simulink model "PhysicalEverSimmer"  (R2026a)
settings: Solver=VariableStepAuto  StopTime=14400
undefined symbols (not defined in the file or in its folder): ES_PackRate_bph, ES_PrepRate_bph, ES_QCRate_bph, ES_Resupply_bph, Fault_T_Cell1, Fault_T_Cell2, Fault_T_Cell3, Recipe_Block_s, Recipe_Count, Resupply_Cutoff_T, Transport_Latency_s, Transport_Rate_bph
(part 2 of 2)

== system PhysicalEverSimmer/ProductionCell1/CellCookVat ==
  in_preppedBatch : Inport  PortName=preppedBatch  Element=flow_bps
  in_directive : Inport  Port=2  PortName=directive  Element=setpoint
  En_Gate_Fault_T_Cell1 : Product
  Gate_Fault_T_Cell1 : Step  Time=Fault_T_Cell1  InitialValue=1  FinalValue=0  SampleTime=0
  StateDbl : DataTypeConversion  OutDataTypeStr=double  SaturateOnIntegerOverflow=off  RndMeth=Floor
  ToLitres : Gain  Gain=1800
  Trm37 : Terminator
  Vat : ModelReference  ModelNameDialog=BehCookVat  UsingDefaultArgumentValue=0,0,0,0,0,0,0,0  SimulationMode=Normal  ModelReferenceVersion=1.8
  cookedSoup_c1 : Constant  Value=0
  cookedSoup_c2 : Constant  Value=0
  statusCook_c1 : Constant
  statusCook_c2 : Constant  Value=0
  out_cookedSoup : Outport  PortName=cookedSoup  Element=batchId
  cookedSoup_el2 : Outport  PortName=cookedSoup  Element=volume_L
  cookedSoup_el3 : Outport  PortName=cookedSoup  Element=temp_C
  cookedSoup_el4 : Outport  PortName=cookedSoup  Element=contamination_ppm
  cookedSoup_el5 : Outport  PortName=cookedSoup  Element=flow_bps
  out_statusCook : Outport  Port=2  PortName=statusCook  Element=unitId
  statusCook_el2 : Outport  Port=2  PortName=statusCook  Element=opState
  statusCook_el3 : Outport  Port=2  PortName=statusCook  Element=faultCode
  statusCook_el4 : Outport  Port=2  PortName=statusCook  Element=power_kW
  statusCook_el5 : Outport  Port=2  PortName=statusCook  Element=health
  wires:
  cookedSoup_c2/1 -> cookedSoup_el4/1
  En_Gate_Fault_T_Cell1/1 -> Vat/2
  statusCook_c1/1 -> out_statusCook/1
  in_directive/1 -> En_Gate_Fault_T_Cell1/1
  statusCook_c2/1 -> statusCook_el3/1
  Vat/5 -> Trm37/1
  Gate_Fault_T_Cell1/1 -> En_Gate_Fault_T_Cell1/2, statusCook_el5/1
  cookedSoup_c1/1 -> out_cookedSoup/1
  ToLitres/1 -> cookedSoup_el2/1
  in_preppedBatch/1 -> Vat/1
  Vat/1 -> cookedSoup_el5/1, ToLitres/1
  Vat/2 -> statusCook_el4/1
  Vat/3 -> cookedSoup_el3/1  "vatTemp_Cell1"
  Vat/4 -> StateDbl/1  "vatState_Cell1"
  StateDbl/1 -> statusCook_el2/1

== system PhysicalEverSimmer/ProductionCell1/CellPackager ==
  in_approvedSoup : Inport  PortName=approvedSoup  Element=flow_bps
  in_directive : Inport  Port=2  PortName=directive  Element=setpoint
  En_Gate_Fault_T_Cell1 : Product
  Gate_Fault_T_Cell1 : Step  Time=Fault_T_Cell1  InitialValue=1  FinalValue=0  SampleTime=0
  Pack : ModelReference  ModelNameDialog=BehPackager  UsingDefaultArgumentValue=0,0  SimulationMode=Normal  ModelReferenceVersion=1.4
  PackDraw : Constant  Value=ES_PackRate_bph/3600
  Surge : ModelReference  ModelNameDialog=BehStorage  UsingDefaultArgumentValue=0,0  SimulationMode=Normal  ModelReferenceVersion=1.3
  Trm44 : Terminator
  Trm45 : Terminator
  sealedContainers_c1 : Constant  Value=0
  sealedContainers_c2 : Constant  Value=0
  sealedContainers_c3 : Constant  Value=365
  statusPack_c1 : Constant
  statusPack_c2 : Constant
  statusPack_c3 : Constant  Value=0
  statusPack_c4 : Constant  Value=12
  out_sealedContainers : Outport  PortName=sealedContainers  Element=batchId
  sealedContainers_el2 : Outport  PortName=sealedContainers  Element=count
  sealedContainers_el3 : Outport  PortName=sealedContainers  Element=sealRating_days
  sealedContainers_el4 : Outport  PortName=sealedContainers  Element=flow_bps
  out_statusPack : Outport  Port=2  PortName=statusPack  Element=unitId
  statusPack_el2 : Outport  Port=2  PortName=statusPack  Element=opState
  statusPack_el3 : Outport  Port=2  PortName=statusPack  Element=faultCode
  statusPack_el4 : Outport  Port=2  PortName=statusPack  Element=power_kW
  statusPack_el5 : Outport  Port=2  PortName=statusPack  Element=health
  wires:
  statusPack_c2/1 -> statusPack_el2/1
  sealedContainers_c3/1 -> sealedContainers_el3/1
  statusPack_c3/1 -> statusPack_el3/1
  sealedContainers_c1/1 -> out_sealedContainers/1
  statusPack_c4/1 -> statusPack_el4/1
  Surge/2 -> Trm44/1
  sealedContainers_c2/1 -> sealedContainers_el2/1
  statusPack_c1/1 -> out_statusPack/1
  Gate_Fault_T_Cell1/1 -> En_Gate_Fault_T_Cell1/2, statusPack_el5/1
  in_directive/1 -> En_Gate_Fault_T_Cell1/1
  in_approvedSoup/1 -> Surge/1
  Pack/1 -> sealedContainers_el4/1
  Surge/3 -> Trm45/1
  PackDraw/1 -> Surge/2
  En_Gate_Fault_T_Cell1/1 -> Pack/2
  Surge/1 -> Pack/1

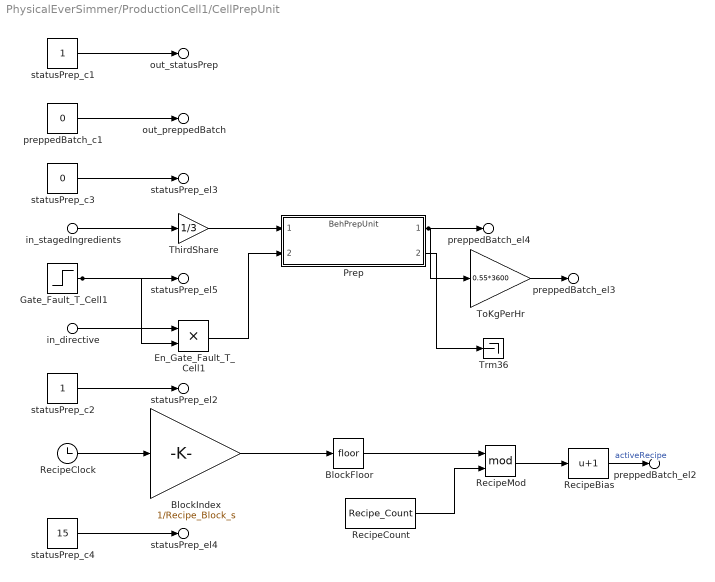
== system PhysicalEverSimmer/ProductionCell1/CellPrepUnit ==
  in_stagedIngredients : Inport  PortName=stagedIngredients  Element=flow_bps
  in_directive : Inport  Port=2  PortName=directive  Element=setpoint
  BlockFloor : Rounding
  BlockIndex : Gain  Gain=1/Recipe_Block_s
  En_Gate_Fault_T_Cell1 : Product
  Gate_Fault_T_Cell1 : Step  Time=Fault_T_Cell1  InitialValue=1  FinalValue=0  SampleTime=0
  Prep : ModelReference  ModelNameDialog=BehPrepUnit  UsingDefaultArgumentValue=0,0  SimulationMode=Normal  ModelReferenceVersion=1.4
  RecipeBias : Bias  Bias=1  SaturateOnIntegerOverflow=off
  RecipeClock : Clock
  RecipeCount : Constant  Value=Recipe_Count
  RecipeMod : Math  Operator=mod
  ThirdShare : Gain  Gain=1/3
  ToKgPerHr : Gain  Gain=0.55*3600
  Trm36 : Terminator
  preppedBatch_c1 : Constant  Value=0
  statusPrep_c1 : Constant
  statusPrep_c2 : Constant
  statusPrep_c3 : Constant  Value=0
  statusPrep_c4 : Constant  Value=15
  out_preppedBatch : Outport  PortName=preppedBatch  Element=batchId
  preppedBatch_el2 : Outport  PortName=preppedBatch  Element=recipeId
  preppedBatch_el3 : Outport  PortName=preppedBatch  Element=mass_kg
  preppedBatch_el4 : Outport  PortName=preppedBatch  Element=flow_bps
  out_statusPrep : Outport  Port=2  PortName=statusPrep  Element=unitId
  statusPrep_el2 : Outport  Port=2  PortName=statusPrep  Element=opState
  statusPrep_el3 : Outport  Port=2  PortName=statusPrep  Element=faultCode
  statusPrep_el4 : Outport  Port=2  PortName=statusPrep  Element=power_kW
  statusPrep_el5 : Outport  Port=2  PortName=statusPrep  Element=health
  wires:
  in_directive/1 -> En_Gate_Fault_T_Cell1/1
  statusPrep_c1/1 -> out_statusPrep/1
  RecipeClock/1 -> BlockIndex/1
  preppedBatch_c1/1 -> out_preppedBatch/1
  statusPrep_c3/1 -> statusPrep_el3/1
  statusPrep_c2/1 -> statusPrep_el2/1
  in_stagedIngredients/1 -> ThirdShare/1
  Gate_Fault_T_Cell1/1 -> En_Gate_Fault_T_Cell1/2, statusPrep_el5/1
  Prep/1 -> preppedBatch_el4/1, ToKgPerHr/1
  statusPrep_c4/1 -> statusPrep_el4/1
  ThirdShare/1 -> Prep/1
  RecipeBias/1 -> preppedBatch_el2/1  "activeRecipe"
  En_Gate_Fault_T_Cell1/1 -> Prep/2
  BlockIndex/1 -> BlockFloor/1
  Prep/2 -> Trm36/1
  BlockFloor/1 -> RecipeMod/1
  RecipeCount/1 -> RecipeMod/2
  ToKgPerHr/1 -> preppedBatch_el3/1
  RecipeMod/1 -> RecipeBias/1

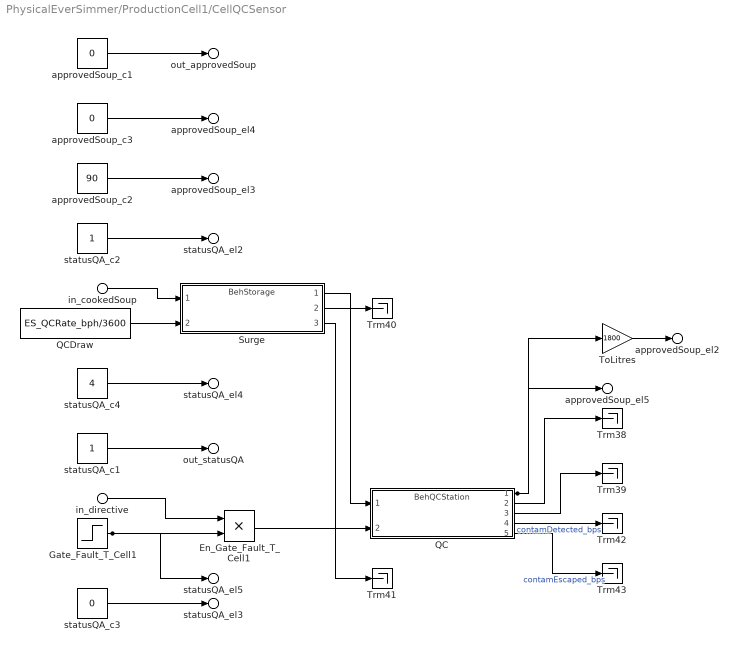
== system PhysicalEverSimmer/ProductionCell1/CellQCSensor ==
  in_cookedSoup : Inport  PortName=cookedSoup  Element=flow_bps
  in_directive : Inport  Port=2  PortName=directive  Element=setpoint
  En_Gate_Fault_T_Cell1 : Product
  Gate_Fault_T_Cell1 : Step  Time=Fault_T_Cell1  InitialValue=1  FinalValue=0  SampleTime=0
  QC : ModelReference  ModelNameDialog=BehQCStation  UsingDefaultArgumentValue=0,0,0,0,0,0  SimulationMode=Normal  ModelReferenceVersion=1.5
  QCDraw : Constant  Value=ES_QCRate_bph/3600
  Surge : ModelReference  ModelNameDialog=BehStorage  UsingDefaultArgumentValue=0,0  SimulationMode=Normal  ModelReferenceVersion=1.3
  ToLitres : Gain  Gain=1800
  Trm{38..43} (6 alike) : Terminator
  approvedSoup_c1 : Constant  Value=0
  approvedSoup_c2 : Constant  Value=90
  approvedSoup_c3 : Constant  Value=0
  statusQA_c1 : Constant
  statusQA_c2 : Constant
  statusQA_c3 : Constant  Value=0
  statusQA_c4 : Constant  Value=4
  out_approvedSoup : Outport  PortName=approvedSoup  Element=batchId
  approvedSoup_el2 : Outport  PortName=approvedSoup  Element=volume_L
  approvedSoup_el3 : Outport  PortName=approvedSoup  Element=temp_C
  approvedSoup_el4 : Outport  PortName=approvedSoup  Element=contamination_ppm
  approvedSoup_el5 : Outport  PortName=approvedSoup  Element=flow_bps
  out_statusQA : Outport  Port=2  PortName=statusQA  Element=unitId
  statusQA_el2 : Outport  Port=2  PortName=statusQA  Element=opState
  statusQA_el3 : Outport  Port=2  PortName=statusQA  Element=faultCode
  statusQA_el4 : Outport  Port=2  PortName=statusQA  Element=power_kW
  statusQA_el5 : Outport  Port=2  PortName=statusQA  Element=health
  wires:
  approvedSoup_c1/1 -> out_approvedSoup/1
  QCDraw/1 -> Surge/2
  approvedSoup_c3/1 -> approvedSoup_el4/1
  Surge/1 -> QC/1
  approvedSoup_c2/1 -> approvedSoup_el3/1
  statusQA_c4/1 -> statusQA_el4/1
  statusQA_c2/1 -> statusQA_el2/1
  in_cookedSoup/1 -> Surge/1
  statusQA_c1/1 -> out_statusQA/1
  in_directive/1 -> En_Gate_Fault_T_Cell1/1
  Gate_Fault_T_Cell1/1 -> En_Gate_Fault_T_Cell1/2, statusQA_el5/1
  En_Gate_Fault_T_Cell1/1 -> QC/2
  statusQA_c3/1 -> statusQA_el3/1
  Surge/2 -> Trm40/1
  QC/4 -> Trm42/1  "contamDetected_bps"
  Surge/3 -> Trm41/1
  QC/1 -> approvedSoup_el5/1, ToLitres/1
  QC/2 -> Trm38/1
  QC/3 -> Trm39/1
  ToLitres/1 -> approvedSoup_el2/1
  QC/5 -> Trm43/1  "contamEscaped_bps"

== system PhysicalEverSimmer/ProductionCell2/CellController ==
  in_directive : Inport  PortName=directive
  statusPrepPwr : Inport  Port=2  PortName=statusPrep  Element=power_kW
  in_statusPrep : Inport  Port=2  PortName=statusPrep  Element=health
  statusCookPwr : Inport  Port=3  PortName=statusCook  Element=power_kW
  in_statusCook : Inport  Port=3  PortName=statusCook  Element=health
  statusQAPwr : Inport  Port=4  PortName=statusQA  Element=power_kW
  in_statusQA : Inport  Port=4  PortName=statusQA  Element=health
  statusPackPwr : Inport  Port=5  PortName=statusPack  Element=power_kW
  in_statusPack : Inport  Port=5  PortName=statusPack  Element=health
  HealthMin : MinMax  Inputs=4
  OwnPower : Constant  Value=2
  PowerSum : Sum  Inputs=+++++
  cellDirective_c1 : Constant  Value=0
  cellDirective_c2 : Constant  Value=0
  cellDirective_c3 : Constant
  statusCell_c1 : Constant  Value=2
  statusCell_c2 : Constant
  statusCell_c3 : Constant  Value=0
  out_cellDirective : Outport  PortName=cellDirective  Element=cmdType
  cellDirective_el2 : Outport  PortName=cellDirective  Element=targetId
  cellDirective_el3 : Outport  PortName=cellDirective  Element=setpoint
  out_statusCell : Outport  Port=2  PortName=statusCell  Element=unitId
  statusCell_el2 : Outport  Port=2  PortName=statusCell  Element=opState
  statusCell_el3 : Outport  Port=2  PortName=statusCell  Element=faultCode
  statusCell_el4 : Outport  Port=2  PortName=statusCell  Element=power_kW
  statusCell_el5 : Outport  Port=2  PortName=statusCell  Element=health
  wires:
  cellDirective_c1/1 -> out_cellDirective/1
  in_statusPack/1 -> HealthMin/4
  cellDirective_c2/1 -> cellDirective_el2/1
  statusCookPwr/1 -> PowerSum/2
  in_statusCook/1 -> HealthMin/2
  statusCell_c2/1 -> statusCell_el2/1
  statusQAPwr/1 -> PowerSum/3
  statusCell_c3/1 -> statusCell_el3/1
  statusPrepPwr/1 -> PowerSum/1
  cellDirective_c3/1 -> cellDirective_el3/1
  statusPackPwr/1 -> PowerSum/4
  OwnPower/1 -> PowerSum/5
  in_statusPrep/1 -> HealthMin/1
  in_statusQA/1 -> HealthMin/3
  statusCell_c1/1 -> out_statusCell/1
  PowerSum/1 -> statusCell_el4/1
  HealthMin/1 -> statusCell_el5/1

== system PhysicalEverSimmer/ProductionCell2/CellCookVat ==
  in_preppedBatch : Inport  PortName=preppedBatch  Element=flow_bps
  in_directive : Inport  Port=2  PortName=directive  Element=setpoint
  En_Gate_Fault_T_Cell2 : Product
  Gate_Fault_T_Cell2 : Step  Time=Fault_T_Cell2  InitialValue=1  FinalValue=0  SampleTime=0
  StateDbl : DataTypeConversion  OutDataTypeStr=double  SaturateOnIntegerOverflow=off  RndMeth=Floor
  ToLitres : Gain  Gain=1800
  Trm47 : Terminator
  Vat : ModelReference  ModelNameDialog=BehCookVat  UsingDefaultArgumentValue=0,0,0,0,0,0,0,0  SimulationMode=Normal  ModelReferenceVersion=1.8
  cookedSoup_c1 : Constant  Value=0
  cookedSoup_c2 : Constant  Value=0
  statusCook_c1 : Constant  Value=2
  statusCook_c2 : Constant  Value=0
  out_cookedSoup : Outport  PortName=cookedSoup  Element=batchId
  cookedSoup_el2 : Outport  PortName=cookedSoup  Element=volume_L
  cookedSoup_el3 : Outport  PortName=cookedSoup  Element=temp_C
  cookedSoup_el4 : Outport  PortName=cookedSoup  Element=contamination_ppm
  cookedSoup_el5 : Outport  PortName=cookedSoup  Element=flow_bps
  out_statusCook : Outport  Port=2  PortName=statusCook  Element=unitId
  statusCook_el2 : Outport  Port=2  PortName=statusCook  Element=opState
  statusCook_el3 : Outport  Port=2  PortName=statusCook  Element=faultCode
  statusCook_el4 : Outport  Port=2  PortName=statusCook  Element=power_kW
  statusCook_el5 : Outport  Port=2  PortName=statusCook  Element=health
  wires:
  cookedSoup_c2/1 -> cookedSoup_el4/1
  Vat/1 -> cookedSoup_el5/1, ToLitres/1
  statusCook_c2/1 -> statusCook_el3/1
  En_Gate_Fault_T_Cell2/1 -> Vat/2
  statusCook_c1/1 -> out_statusCook/1
  cookedSoup_c1/1 -> out_cookedSoup/1
  Gate_Fault_T_Cell2/1 -> statusCook_el5/1, En_Gate_Fault_T_Cell2/2
  in_directive/1 -> En_Gate_Fault_T_Cell2/1
  in_preppedBatch/1 -> Vat/1
  Vat/2 -> statusCook_el4/1
  Vat/3 -> cookedSoup_el3/1
  Vat/4 -> StateDbl/1
  Vat/5 -> Trm47/1
  ToLitres/1 -> cookedSoup_el2/1
  StateDbl/1 -> statusCook_el2/1

== system PhysicalEverSimmer/ProductionCell2/CellPackager ==
  in_approvedSoup : Inport  PortName=approvedSoup  Element=flow_bps
  in_directive : Inport  Port=2  PortName=directive  Element=setpoint
  En_Gate_Fault_T_Cell2 : Product
  Gate_Fault_T_Cell2 : Step  Time=Fault_T_Cell2  InitialValue=1  FinalValue=0  SampleTime=0
  Pack : ModelReference  ModelNameDialog=BehPackager  UsingDefaultArgumentValue=0,0  SimulationMode=Normal  ModelReferenceVersion=1.4
  PackDraw : Constant  Value=ES_PackRate_bph/3600
  Surge : ModelReference  ModelNameDialog=BehStorage  UsingDefaultArgumentValue=0,0  SimulationMode=Normal  ModelReferenceVersion=1.3
  Trm54 : Terminator
  Trm55 : Terminator
  sealedContainers_c1 : Constant  Value=0
  sealedContainers_c2 : Constant  Value=0
  sealedContainers_c3 : Constant  Value=365
  statusPack_c1 : Constant
  statusPack_c2 : Constant
  statusPack_c3 : Constant  Value=0
  statusPack_c4 : Constant  Value=12
  out_sealedContainers : Outport  PortName=sealedContainers  Element=batchId
  sealedContainers_el2 : Outport  PortName=sealedContainers  Element=count
  sealedContainers_el3 : Outport  PortName=sealedContainers  Element=sealRating_days
  sealedContainers_el4 : Outport  PortName=sealedContainers  Element=flow_bps
  out_statusPack : Outport  Port=2  PortName=statusPack  Element=unitId
  statusPack_el2 : Outport  Port=2  PortName=statusPack  Element=opState
  statusPack_el3 : Outport  Port=2  PortName=statusPack  Element=faultCode
  statusPack_el4 : Outport  Port=2  PortName=statusPack  Element=power_kW
  statusPack_el5 : Outport  Port=2  PortName=statusPack  Element=health
  wires:
  sealedContainers_c1/1 -> out_sealedContainers/1
  statusPack_c2/1 -> statusPack_el2/1
  statusPack_c1/1 -> out_statusPack/1
  sealedContainers_c3/1 -> sealedContainers_el3/1
  statusPack_c4/1 -> statusPack_el4/1
  statusPack_c3/1 -> statusPack_el3/1
  Gate_Fault_T_Cell2/1 -> statusPack_el5/1, En_Gate_Fault_T_Cell2/2
  Surge/1 -> Pack/1
  in_directive/1 -> En_Gate_Fault_T_Cell2/1
  in_approvedSoup/1 -> Surge/1
  PackDraw/1 -> Surge/2
  sealedContainers_c2/1 -> sealedContainers_el2/1
  En_Gate_Fault_T_Cell2/1 -> Pack/2
  Surge/2 -> Trm54/1
  Surge/3 -> Trm55/1
  Pack/1 -> sealedContainers_el4/1

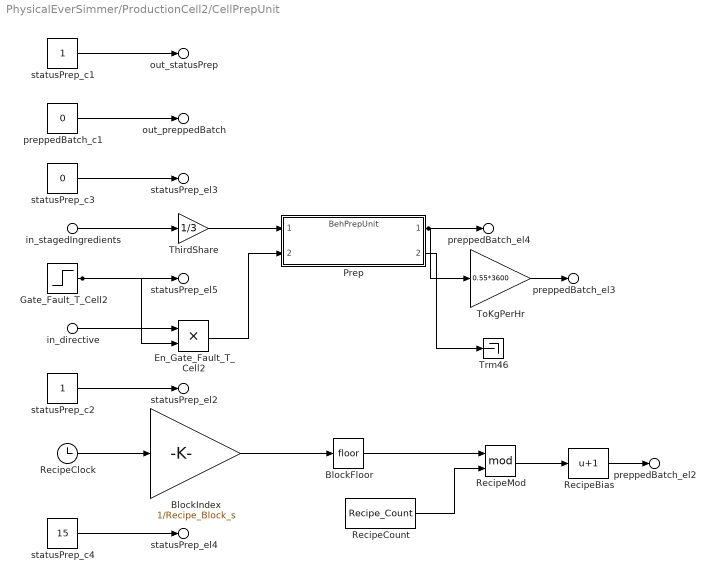
== system PhysicalEverSimmer/ProductionCell2/CellPrepUnit ==
  in_stagedIngredients : Inport  PortName=stagedIngredients  Element=flow_bps
  in_directive : Inport  Port=2  PortName=directive  Element=setpoint
  BlockFloor : Rounding
  BlockIndex : Gain  Gain=1/Recipe_Block_s
  En_Gate_Fault_T_Cell2 : Product
  Gate_Fault_T_Cell2 : Step  Time=Fault_T_Cell2  InitialValue=1  FinalValue=0  SampleTime=0
  Prep : ModelReference  ModelNameDialog=BehPrepUnit  UsingDefaultArgumentValue=0,0  SimulationMode=Normal  ModelReferenceVersion=1.4
  RecipeBias : Bias  Bias=1  SaturateOnIntegerOverflow=off
  RecipeClock : Clock
  RecipeCount : Constant  Value=Recipe_Count
  RecipeMod : Math  Operator=mod
  ThirdShare : Gain  Gain=1/3
  ToKgPerHr : Gain  Gain=0.55*3600
  Trm46 : Terminator
  preppedBatch_c1 : Constant  Value=0
  statusPrep_c1 : Constant
  statusPrep_c2 : Constant
  statusPrep_c3 : Constant  Value=0
  statusPrep_c4 : Constant  Value=15
  out_preppedBatch : Outport  PortName=preppedBatch  Element=batchId
  preppedBatch_el2 : Outport  PortName=preppedBatch  Element=recipeId
  preppedBatch_el3 : Outport  PortName=preppedBatch  Element=mass_kg
  preppedBatch_el4 : Outport  PortName=preppedBatch  Element=flow_bps
  out_statusPrep : Outport  Port=2  PortName=statusPrep  Element=unitId
  statusPrep_el2 : Outport  Port=2  PortName=statusPrep  Element=opState
  statusPrep_el3 : Outport  Port=2  PortName=statusPrep  Element=faultCode
  statusPrep_el4 : Outport  Port=2  PortName=statusPrep  Element=power_kW
  statusPrep_el5 : Outport  Port=2  PortName=statusPrep  Element=health
  wires:
  statusPrep_c1/1 -> out_statusPrep/1
  preppedBatch_c1/1 -> out_preppedBatch/1
  statusPrep_c3/1 -> statusPrep_el3/1
  in_directive/1 -> En_Gate_Fault_T_Cell2/1
  in_stagedIngredients/1 -> ThirdShare/1
  BlockFloor/1 -> RecipeMod/1
  Gate_Fault_T_Cell2/1 -> En_Gate_Fault_T_Cell2/2, statusPrep_el5/1
  statusPrep_c2/1 -> statusPrep_el2/1
  RecipeClock/1 -> BlockIndex/1
  statusPrep_c4/1 -> statusPrep_el4/1
  ThirdShare/1 -> Prep/1
  En_Gate_Fault_T_Cell2/1 -> Prep/2
  BlockIndex/1 -> BlockFloor/1
  Prep/1 -> preppedBatch_el4/1, ToKgPerHr/1
  Prep/2 -> Trm46/1
  RecipeCount/1 -> RecipeMod/2
  ToKgPerHr/1 -> preppedBatch_el3/1
  RecipeMod/1 -> RecipeBias/1
  RecipeBias/1 -> preppedBatch_el2/1

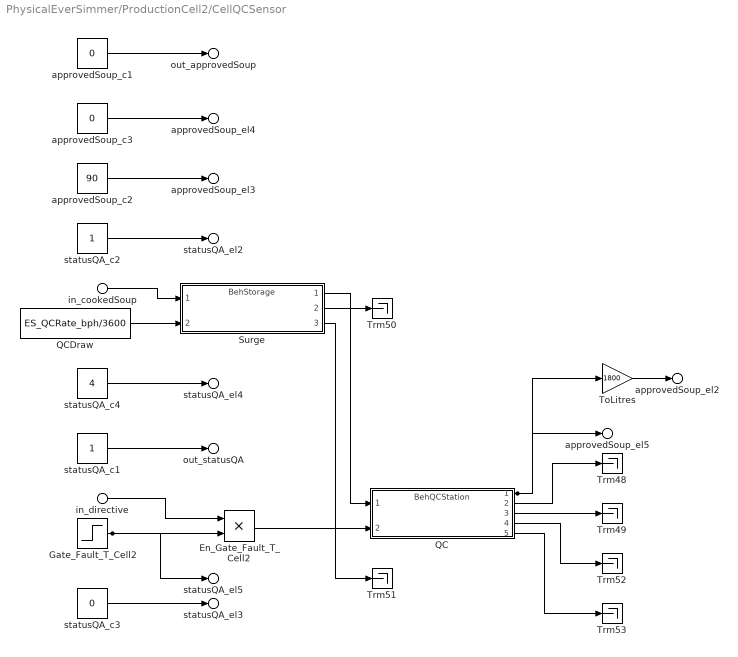
== system PhysicalEverSimmer/ProductionCell2/CellQCSensor ==
  in_cookedSoup : Inport  PortName=cookedSoup  Element=flow_bps
  in_directive : Inport  Port=2  PortName=directive  Element=setpoint
  En_Gate_Fault_T_Cell2 : Product
  Gate_Fault_T_Cell2 : Step  Time=Fault_T_Cell2  InitialValue=1  FinalValue=0  SampleTime=0
  QC : ModelReference  ModelNameDialog=BehQCStation  UsingDefaultArgumentValue=0,0,0,0,0,0  SimulationMode=Normal  ModelReferenceVersion=1.5
  QCDraw : Constant  Value=ES_QCRate_bph/3600
  Surge : ModelReference  ModelNameDialog=BehStorage  UsingDefaultArgumentValue=0,0  SimulationMode=Normal  ModelReferenceVersion=1.3
  ToLitres : Gain  Gain=1800
  Trm{48..53} (6 alike) : Terminator
  approvedSoup_c1 : Constant  Value=0
  approvedSoup_c2 : Constant  Value=90
  approvedSoup_c3 : Constant  Value=0
  statusQA_c1 : Constant
  statusQA_c2 : Constant
  statusQA_c3 : Constant  Value=0
  statusQA_c4 : Constant  Value=4
  out_approvedSoup : Outport  PortName=approvedSoup  Element=batchId
  approvedSoup_el2 : Outport  PortName=approvedSoup  Element=volume_L
  approvedSoup_el3 : Outport  PortName=approvedSoup  Element=temp_C
  approvedSoup_el4 : Outport  PortName=approvedSoup  Element=contamination_ppm
  approvedSoup_el5 : Outport  PortName=approvedSoup  Element=flow_bps
  out_statusQA : Outport  Port=2  PortName=statusQA  Element=unitId
  statusQA_el2 : Outport  Port=2  PortName=statusQA  Element=opState
  statusQA_el3 : Outport  Port=2  PortName=statusQA  Element=faultCode
  statusQA_el4 : Outport  Port=2  PortName=statusQA  Element=power_kW
  statusQA_el5 : Outport  Port=2  PortName=statusQA  Element=health
  wires:
  approvedSoup_c1/1 -> out_approvedSoup/1
  statusQA_c4/1 -> statusQA_el4/1
  approvedSoup_c3/1 -> approvedSoup_el4/1
  ToLitres/1 -> approvedSoup_el2/1
  QC/2 -> Trm48/1
  approvedSoup_c2/1 -> approvedSoup_el3/1
  statusQA_c3/1 -> statusQA_el3/1
  QCDraw/1 -> Surge/2
  statusQA_c2/1 -> statusQA_el2/1
  in_cookedSoup/1 -> Surge/1
  statusQA_c1/1 -> out_statusQA/1
  in_directive/1 -> En_Gate_Fault_T_Cell2/1
  Gate_Fault_T_Cell2/1 -> En_Gate_Fault_T_Cell2/2, statusQA_el5/1
  QC/4 -> Trm52/1
  Surge/1 -> QC/1
  Surge/2 -> Trm50/1
  Surge/3 -> Trm51/1
  En_Gate_Fault_T_Cell2/1 -> QC/2
  QC/1 -> approvedSoup_el5/1, ToLitres/1
  QC/3 -> Trm49/1
  QC/5 -> Trm53/1

== system PhysicalEverSimmer/ProductionCell3/CellController ==
  in_directive : Inport  PortName=directive
  statusPrepPwr : Inport  Port=2  PortName=statusPrep  Element=power_kW
  in_statusPrep : Inport  Port=2  PortName=statusPrep  Element=health
  statusCookPwr : Inport  Port=3  PortName=statusCook  Element=power_kW
  in_statusCook : Inport  Port=3  PortName=statusCook  Element=health
  statusQAPwr : Inport  Port=4  PortName=statusQA  Element=power_kW
  in_statusQA : Inport  Port=4  PortName=statusQA  Element=health
  statusPackPwr : Inport  Port=5  PortName=statusPack  Element=power_kW
  in_statusPack : Inport  Port=5  PortName=statusPack  Element=health
  HealthMin : MinMax  Inputs=4
  OwnPower : Constant  Value=2
  PowerSum : Sum  Inputs=+++++
  cellDirective_c1 : Constant  Value=0
  cellDirective_c2 : Constant  Value=0
  cellDirective_c3 : Constant
  statusCell_c1 : Constant  Value=3
  statusCell_c2 : Constant
  statusCell_c3 : Constant  Value=0
  out_cellDirective : Outport  PortName=cellDirective  Element=cmdType
  cellDirective_el2 : Outport  PortName=cellDirective  Element=targetId
  cellDirective_el3 : Outport  PortName=cellDirective  Element=setpoint
  out_statusCell : Outport  Port=2  PortName=statusCell  Element=unitId
  statusCell_el2 : Outport  Port=2  PortName=statusCell  Element=opState
  statusCell_el3 : Outport  Port=2  PortName=statusCell  Element=faultCode
  statusCell_el4 : Outport  Port=2  PortName=statusCell  Element=power_kW
  statusCell_el5 : Outport  Port=2  PortName=statusCell  Element=health
  wires:
  statusCell_c2/1 -> statusCell_el2/1
  cellDirective_c1/1 -> out_cellDirective/1
  statusQAPwr/1 -> PowerSum/3
  HealthMin/1 -> statusCell_el5/1
  statusCell_c3/1 -> statusCell_el3/1
  cellDirective_c2/1 -> cellDirective_el2/1
  statusPrepPwr/1 -> PowerSum/1
  cellDirective_c3/1 -> cellDirective_el3/1
  statusCookPwr/1 -> PowerSum/2
  statusPackPwr/1 -> PowerSum/4
  OwnPower/1 -> PowerSum/5
  in_statusPrep/1 -> HealthMin/1
  in_statusPack/1 -> HealthMin/4
  in_statusCook/1 -> HealthMin/2
  in_statusQA/1 -> HealthMin/3
  statusCell_c1/1 -> out_statusCell/1
  PowerSum/1 -> statusCell_el4/1

== system PhysicalEverSimmer/ProductionCell3/CellCookVat ==
  in_preppedBatch : Inport  PortName=preppedBatch  Element=flow_bps
  in_directive : Inport  Port=2  PortName=directive  Element=setpoint
  En_Gate_Fault_T_Cell3 : Product
  Gate_Fault_T_Cell3 : Step  Time=Fault_T_Cell3  InitialValue=1  FinalValue=0  SampleTime=0
  StateDbl : DataTypeConversion  OutDataTypeStr=double  SaturateOnIntegerOverflow=off  RndMeth=Floor
  ToLitres : Gain  Gain=1800
  Trm57 : Terminator
  Vat : ModelReference  ModelNameDialog=BehCookVat  UsingDefaultArgumentValue=0,0,0,0,0,0,0,0  SimulationMode=Normal  ModelReferenceVersion=1.8
  cookedSoup_c1 : Constant  Value=0
  cookedSoup_c2 : Constant  Value=0
  statusCook_c1 : Constant  Value=3
  statusCook_c2 : Constant  Value=0
  out_cookedSoup : Outport  PortName=cookedSoup  Element=batchId
  cookedSoup_el2 : Outport  PortName=cookedSoup  Element=volume_L
  cookedSoup_el3 : Outport  PortName=cookedSoup  Element=temp_C
  cookedSoup_el4 : Outport  PortName=cookedSoup  Element=contamination_ppm
  cookedSoup_el5 : Outport  PortName=cookedSoup  Element=flow_bps
  out_statusCook : Outport  Port=2  PortName=statusCook  Element=unitId
  statusCook_el2 : Outport  Port=2  PortName=statusCook  Element=opState
  statusCook_el3 : Outport  Port=2  PortName=statusCook  Element=faultCode
  statusCook_el4 : Outport  Port=2  PortName=statusCook  Element=power_kW
  statusCook_el5 : Outport  Port=2  PortName=statusCook  Element=health
  wires:
  En_Gate_Fault_T_Cell3/1 -> Vat/2
  cookedSoup_c2/1 -> cookedSoup_el4/1
  Gate_Fault_T_Cell3/1 -> En_Gate_Fault_T_Cell3/2, statusCook_el5/1
  statusCook_c2/1 -> statusCook_el3/1
  in_preppedBatch/1 -> Vat/1
  statusCook_c1/1 -> out_statusCook/1
  cookedSoup_c1/1 -> out_cookedSoup/1
  in_directive/1 -> En_Gate_Fault_T_Cell3/1
  Vat/1 -> cookedSoup_el5/1, ToLitres/1
  Vat/2 -> statusCook_el4/1
  Vat/3 -> cookedSoup_el3/1
  Vat/4 -> StateDbl/1
  Vat/5 -> Trm57/1
  ToLitres/1 -> cookedSoup_el2/1
  StateDbl/1 -> statusCook_el2/1

== system PhysicalEverSimmer/ProductionCell3/CellPackager ==
  in_approvedSoup : Inport  PortName=approvedSoup  Element=flow_bps
  in_directive : Inport  Port=2  PortName=directive  Element=setpoint
  En_Gate_Fault_T_Cell3 : Product
  Gate_Fault_T_Cell3 : Step  Time=Fault_T_Cell3  InitialValue=1  FinalValue=0  SampleTime=0
  Pack : ModelReference  ModelNameDialog=BehPackager  UsingDefaultArgumentValue=0,0  SimulationMode=Normal  ModelReferenceVersion=1.4
  PackDraw : Constant  Value=ES_PackRate_bph/3600
  Surge : ModelReference  ModelNameDialog=BehStorage  UsingDefaultArgumentValue=0,0  SimulationMode=Normal  ModelReferenceVersion=1.3
  Trm64 : Terminator
  Trm65 : Terminator
  sealedContainers_c1 : Constant  Value=0
  sealedContainers_c2 : Constant  Value=0
  sealedContainers_c3 : Constant  Value=365
  statusPack_c1 : Constant
  statusPack_c2 : Constant
  statusPack_c3 : Constant  Value=0
  statusPack_c4 : Constant  Value=12
  out_sealedContainers : Outport  PortName=sealedContainers  Element=batchId
  sealedContainers_el2 : Outport  PortName=sealedContainers  Element=count
  sealedContainers_el3 : Outport  PortName=sealedContainers  Element=sealRating_days
  sealedContainers_el4 : Outport  PortName=sealedContainers  Element=flow_bps
  out_statusPack : Outport  Port=2  PortName=statusPack  Element=unitId
  statusPack_el2 : Outport  Port=2  PortName=statusPack  Element=opState
  statusPack_el3 : Outport  Port=2  PortName=statusPack  Element=faultCode
  statusPack_el4 : Outport  Port=2  PortName=statusPack  Element=power_kW
  statusPack_el5 : Outport  Port=2  PortName=statusPack  Element=health
  wires:
  statusPack_c2/1 -> statusPack_el2/1
  sealedContainers_c3/1 -> sealedContainers_el3/1
  statusPack_c4/1 -> statusPack_el4/1
  statusPack_c1/1 -> out_statusPack/1
  in_directive/1 -> En_Gate_Fault_T_Cell3/1
  sealedContainers_c1/1 -> out_sealedContainers/1
  statusPack_c3/1 -> statusPack_el3/1
  Gate_Fault_T_Cell3/1 -> En_Gate_Fault_T_Cell3/2, statusPack_el5/1
  in_approvedSoup/1 -> Surge/1
  En_Gate_Fault_T_Cell3/1 -> Pack/2
  PackDraw/1 -> Surge/2
  sealedContainers_c2/1 -> sealedContainers_el2/1
  Surge/1 -> Pack/1
  Surge/2 -> Trm64/1
  Surge/3 -> Trm65/1
  Pack/1 -> sealedContainers_el4/1

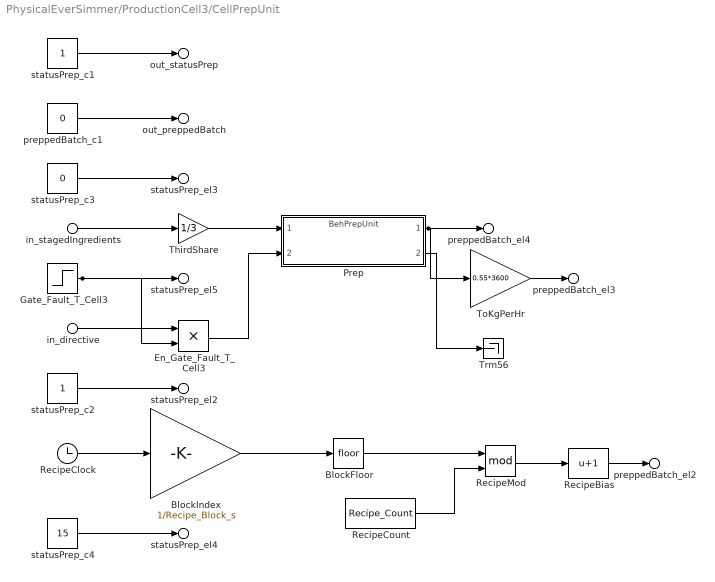
== system PhysicalEverSimmer/ProductionCell3/CellPrepUnit ==
  in_stagedIngredients : Inport  PortName=stagedIngredients  Element=flow_bps
  in_directive : Inport  Port=2  PortName=directive  Element=setpoint
  BlockFloor : Rounding
  BlockIndex : Gain  Gain=1/Recipe_Block_s
  En_Gate_Fault_T_Cell3 : Product
  Gate_Fault_T_Cell3 : Step  Time=Fault_T_Cell3  InitialValue=1  FinalValue=0  SampleTime=0
  Prep : ModelReference  ModelNameDialog=BehPrepUnit  UsingDefaultArgumentValue=0,0  SimulationMode=Normal  ModelReferenceVersion=1.4
  RecipeBias : Bias  Bias=1  SaturateOnIntegerOverflow=off
  RecipeClock : Clock
  RecipeCount : Constant  Value=Recipe_Count
  RecipeMod : Math  Operator=mod
  ThirdShare : Gain  Gain=1/3
  ToKgPerHr : Gain  Gain=0.55*3600
  Trm56 : Terminator
  preppedBatch_c1 : Constant  Value=0
  statusPrep_c1 : Constant
  statusPrep_c2 : Constant
  statusPrep_c3 : Constant  Value=0
  statusPrep_c4 : Constant  Value=15
  out_preppedBatch : Outport  PortName=preppedBatch  Element=batchId
  preppedBatch_el2 : Outport  PortName=preppedBatch  Element=recipeId
  preppedBatch_el3 : Outport  PortName=preppedBatch  Element=mass_kg
  preppedBatch_el4 : Outport  PortName=preppedBatch  Element=flow_bps
  out_statusPrep : Outport  Port=2  PortName=statusPrep  Element=unitId
  statusPrep_el2 : Outport  Port=2  PortName=statusPrep  Element=opState
  statusPrep_el3 : Outport  Port=2  PortName=statusPrep  Element=faultCode
  statusPrep_el4 : Outport  Port=2  PortName=statusPrep  Element=power_kW
  statusPrep_el5 : Outport  Port=2  PortName=statusPrep  Element=health
  wires:
  in_directive/1 -> En_Gate_Fault_T_Cell3/1
  statusPrep_c1/1 -> out_statusPrep/1
  RecipeClock/1 -> BlockIndex/1
  in_stagedIngredients/1 -> ThirdShare/1
  preppedBatch_c1/1 -> out_preppedBatch/1
  Gate_Fault_T_Cell3/1 -> En_Gate_Fault_T_Cell3/2, statusPrep_el5/1
  statusPrep_c3/1 -> statusPrep_el3/1
  statusPrep_c2/1 -> statusPrep_el2/1
  statusPrep_c4/1 -> statusPrep_el4/1
  ThirdShare/1 -> Prep/1
  En_Gate_Fault_T_Cell3/1 -> Prep/2
  BlockIndex/1 -> BlockFloor/1
  Prep/1 -> preppedBatch_el4/1, ToKgPerHr/1
  Prep/2 -> Trm56/1
  BlockFloor/1 -> RecipeMod/1
  RecipeCount/1 -> RecipeMod/2
  ToKgPerHr/1 -> preppedBatch_el3/1
  RecipeMod/1 -> RecipeBias/1
  RecipeBias/1 -> preppedBatch_el2/1

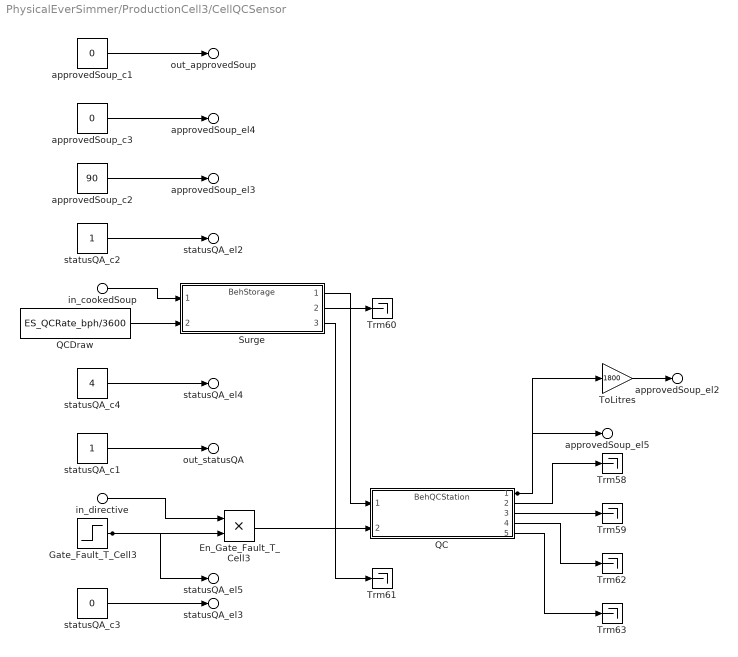
== system PhysicalEverSimmer/ProductionCell3/CellQCSensor ==
  in_cookedSoup : Inport  PortName=cookedSoup  Element=flow_bps
  in_directive : Inport  Port=2  PortName=directive  Element=setpoint
  En_Gate_Fault_T_Cell3 : Product
  Gate_Fault_T_Cell3 : Step  Time=Fault_T_Cell3  InitialValue=1  FinalValue=0  SampleTime=0
  QC : ModelReference  ModelNameDialog=BehQCStation  UsingDefaultArgumentValue=0,0,0,0,0,0  SimulationMode=Normal  ModelReferenceVersion=1.5
  QCDraw : Constant  Value=ES_QCRate_bph/3600
  Surge : ModelReference  ModelNameDialog=BehStorage  UsingDefaultArgumentValue=0,0  SimulationMode=Normal  ModelReferenceVersion=1.3
  ToLitres : Gain  Gain=1800
  Trm{58..63} (6 alike) : Terminator
  approvedSoup_c1 : Constant  Value=0
  approvedSoup_c2 : Constant  Value=90
  approvedSoup_c3 : Constant  Value=0
  statusQA_c1 : Constant
  statusQA_c2 : Constant
  statusQA_c3 : Constant  Value=0
  statusQA_c4 : Constant  Value=4
  out_approvedSoup : Outport  PortName=approvedSoup  Element=batchId
  approvedSoup_el2 : Outport  PortName=approvedSoup  Element=volume_L
  approvedSoup_el3 : Outport  PortName=approvedSoup  Element=temp_C
  approvedSoup_el4 : Outport  PortName=approvedSoup  Element=contamination_ppm
  approvedSoup_el5 : Outport  PortName=approvedSoup  Element=flow_bps
  out_statusQA : Outport  Port=2  PortName=statusQA  Element=unitId
  statusQA_el2 : Outport  Port=2  PortName=statusQA  Element=opState
  statusQA_el3 : Outport  Port=2  PortName=statusQA  Element=faultCode
  statusQA_el4 : Outport  Port=2  PortName=statusQA  Element=power_kW
  statusQA_el5 : Outport  Port=2  PortName=statusQA  Element=health
  wires:
  statusQA_c2/1 -> statusQA_el2/1
  approvedSoup_c1/1 -> out_approvedSoup/1
  statusQA_c4/1 -> statusQA_el4/1
  approvedSoup_c3/1 -> approvedSoup_el4/1
  approvedSoup_c2/1 -> approvedSoup_el3/1
  in_cookedSoup/1 -> Surge/1
  QCDraw/1 -> Surge/2
  statusQA_c1/1 -> out_statusQA/1
  in_directive/1 -> En_Gate_Fault_T_Cell3/1
  Gate_Fault_T_Cell3/1 -> En_Gate_Fault_T_Cell3/2, statusQA_el5/1
  statusQA_c3/1 -> statusQA_el3/1
  Surge/1 -> QC/1
  Surge/2 -> Trm60/1
  Surge/3 -> Trm61/1
  En_Gate_Fault_T_Cell3/1 -> QC/2
  QC/1 -> approvedSoup_el5/1, ToLitres/1
  QC/2 -> Trm58/1
  QC/3 -> Trm59/1
  QC/4 -> Trm62/1
  QC/5 -> Trm63/1
  ToLitres/1 -> approvedSoup_el2/1
